simulink model "ashepwm_N3"  (R2017b)
settings: Solver=ode3  StartTime=0.0  StopTime=1  FixedStep=5e-6  MaxStep=1e-4  RelTol=1e-3
libraries: powerlib x12, simulink x1
settings Model: Creator=zsrx  LastModifiedBy=zsrx

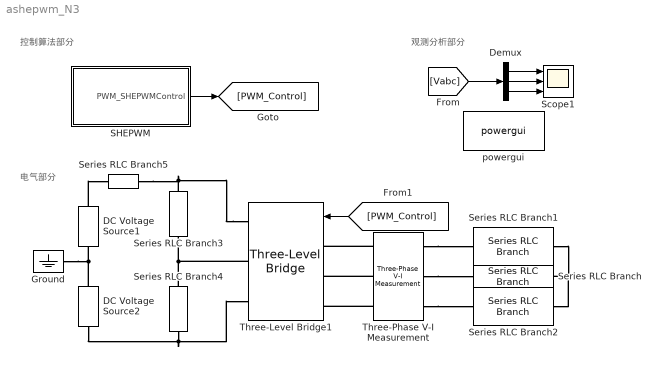
== system ashepwm_N3 ==
  note: 观测分析部分
  note: 控制算法部分
  note: 电气部分
  DC Voltage Source1 : powerlib/Electrical Sources/DC Voltage Source  Amplitude=345  Measurements=Voltage
  DC Voltage Source2 : powerlib/Electrical Sources/DC Voltage Source  Amplitude=345  Measurements=Voltage
  Demux : Demux  Outputs=3
  Ground : powerlib/Elements/Ground  LConnTagsString=a
  SHEPWM : Subsystem
  Scope1 : Scope  NumInputPorts=3
  Series RLC Branch : powerlib/Elements/Series RLC Branch  LConnTagsString=__new0  RConnTagsString=__new0  BranchType=R  Resistance=20  Inductance=1e-3  SetiL0=off  InitialCurrent=0  Capacitance=1e-6  Setx0=off  InitialVoltage=0  Measurements=None
  Series RLC Branch1 : powerlib/Elements/Series RLC Branch  LConnTagsString=__new0  RConnTagsString=__new0  BranchType=R  Resistance=20  Inductance=1e-3  SetiL0=off  InitialCurrent=0  Capacitance=1e-6  Setx0=off  InitialVoltage=0  Measurements=None
  Series RLC Branch2 : powerlib/Elements/Series RLC Branch  LConnTagsString=__new0  RConnTagsString=__new0  BranchType=R  Resistance=20  Inductance=1e-3  SetiL0=off  InitialCurrent=0  Capacitance=1e-6  Setx0=off  InitialVoltage=0  Measurements=None
  Series RLC Branch3 : powerlib/Elements/Series RLC Branch  LConnTagsString=__new0  RConnTagsString=__new0  BranchType=C  Resistance=20  Inductance=1e-3  SetiL0=off  InitialCurrent=0  Capacitance=9000e-6  Setx0=off  InitialVoltage=0  Measurements=None
  Series RLC Branch4 : powerlib/Elements/Series RLC Branch  LConnTagsString=__new0  RConnTagsString=__new0  BranchType=C  Resistance=20  Inductance=1e-3  SetiL0=off  InitialCurrent=0  Capacitance=9000e-6  Setx0=off  InitialVoltage=0  Measurements=None
  Series RLC Branch5 : powerlib/Elements/Series RLC Branch  LConnTagsString=__new0  RConnTagsString=__new0  BranchType=R  Resistance=0.001  Inductance=1e-3  SetiL0=off  InitialCurrent=0  Capacitance=1e-6  Setx0=off  InitialVoltage=0  Measurements=None
  Three-Level Bridge1 : powerlib/Power Electronics/Three-Level Bridge  Arms=3  SnubberResistance=1e5  SbubberCapacitance=inf  Device=GTO / Diodes  Ron=1e-3  ForwardVoltages="[  0  0  ]"  Measurements=None
      settings: SourceProductName=Simscape Power Systems  SourceProductBaseCode=PS
  Three-Phase V-I Measurement : powerlib/Measurements/Three-Phase V-I Measurement  VoltageMeasurement=phase-to-ground  SetLabelV=on  LabelV=Vabc  Vpu=off  VpuLL=off  CurrentMeasurement=yes  SetLabelI=on  LabelI=Iabc  Ipu=off  Pbase=100e6  Vbase=500e3  OutputType=Complex  PhasorSimulation=off  PSBequivalent=0
  powergui : powerlib/powergui  Priority=1  SimulationMode=Discrete  SampleTime=5e-6  frequency=60  Iterations=50  frequencyindice=0  Pbase=100e6  ErrMax=1e-4  UnitsV=kV  UnitsW=MW  buscounter=0  FunctionMessages=off  echomessages=off  EnableUseOfTLC=off  CurrentSourceSwitches=off  DisableSnubberDevices=off  DisableRonSwitches=off  DisableVfSwitches=off  DisplayEquations=off  SolverType=Tustin/Backward Euler (TBE)  Interpol=off  ExternalGateDelay=off  methode=off  Ts=100  x0status=blocks  SPID=off  SwTol=0  HookPort=off  RestoreLinks=warning  ResistiveCurrentMeasurement=off  Frange=[0:2:500]  Ylog=off  Xlog=on  ShowGrid=off  save=off  variable=ZData  structure=ScopeData1  ZoomFFT=off  StartTime=0.5  cycles=1  DisplayStyle=2  fundamental=50  FreqAxis=off  MaxFrequency=1000  frequencyindicesteady=1  RmsSteady=1  display=off
  wires:
  SHEPWM/1(PWM_SHEPWMControl) -> [PWM_Control]
  [PWM_Control] -> Three-Level Bridge1/1
  Demux/1 -> Scope1/1
  [Vabc] -> Demux/1
  Demux/2 -> Scope1/2
  Demux/3 -> Scope1/3
  connections:
  DC Voltage Source2/RConn1 -- Ground/LConn1 -- DC Voltage Source1/LConn1
  Three-Level Bridge1/RConn1 -- Series RLC Branch5/LConn1 -- Series RLC Branch3/LConn1
  DC Voltage Source2/LConn1 -- Series RLC Branch4/RConn1 -- Three-Level Bridge1/RConn3
  Series RLC Branch1/RConn1 -- Series RLC Branch2/RConn1 -- Series RLC Branch/RConn1
  Series RLC Branch4/LConn1 -- Three-Level Bridge1/RConn2 -- Series RLC Branch3/RConn1
  DC Voltage Source1/RConn1 -- Series RLC Branch5/RConn1
  Three-Phase V-I Measurement/LConn1 -- Three-Level Bridge1/LConn1
  Three-Phase V-I Measurement/LConn2 -- Three-Level Bridge1/LConn2
  Three-Phase V-I Measurement/LConn3 -- Three-Level Bridge1/LConn3
  Three-Phase V-I Measurement/RConn3 -- Series RLC Branch2/LConn1
  Three-Phase V-I Measurement/RConn2 -- Series RLC Branch/LConn1
  Three-Phase V-I Measurement/RConn1 -- Series RLC Branch1/LConn1

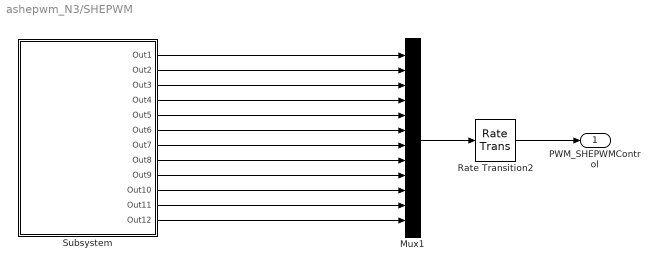
== system ashepwm_N3/SHEPWM ==
  Mux1 : Mux  Inputs=12
  Rate Transition2 : RateTransition  OutPortSampleTime=5e-6
  Subsystem : Subsystem
  PWM_SHEPWMControl : Outport
  wires:
  Subsystem/1(Out1) -> Mux1/1
  Subsystem/9(Out9) -> Mux1/9
  Subsystem/10(Out10) -> Mux1/10
  Subsystem/11(Out11) -> Mux1/11
  Subsystem/12(Out12) -> Mux1/12
  Mux1/1 -> Rate Transition2/1
  Subsystem/3(Out3) -> Mux1/3
  Subsystem/4(Out4) -> Mux1/4
  Subsystem/2(Out2) -> Mux1/2
  Subsystem/5(Out5) -> Mux1/5
  Subsystem/6(Out6) -> Mux1/6
  Subsystem/7(Out7) -> Mux1/7
  Subsystem/8(Out8) -> Mux1/8
  Rate Transition2/1 -> PWM_SHEPWMControl/1

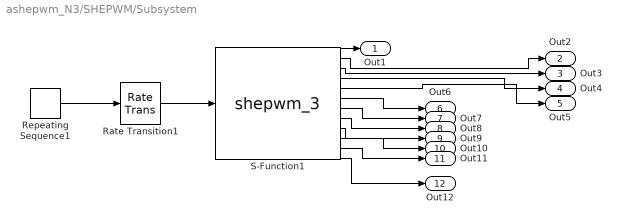
== system ashepwm_N3/SHEPWM/Subsystem ==
  Rate Transition1 : RateTransition  OutPortSampleTime=5e-5
  Repeating Sequence1 : simulink/Sources/Repeating Sequence  rep_seq_t=[0 0.02]  rep_seq_y=[0 6.2831852]
  S-Function1 : S-Function  FunctionName=shepwm_3  SFunctionDeploymentMode=off  EnableBusSupport=off
  Out1 : Outport
  Out2 : Outport  Port=2
  Out3 : Outport  Port=3
  Out4 : Outport  Port=4
  Out5 : Outport  Port=5
  Out6 : Outport  Port=6
  Out7 : Outport  Port=7
  Out8 : Outport  Port=8
  Out9 : Outport  Port=9
  Out10 : Outport  Port=10
  Out11 : Outport  Port=11
  Out12 : Outport  Port=12
  wires:
  S-Function1/1 -> Out1/1
  Repeating Sequence1/1 -> Rate Transition1/1
  Rate Transition1/1 -> S-Function1/1
  S-Function1/2 -> Out2/1
  S-Function1/4 -> Out4/1
  S-Function1/5 -> Out5/1
  S-Function1/3 -> Out3/1
  S-Function1/6 -> Out6/1
  S-Function1/7 -> Out7/1
  S-Function1/8 -> Out8/1
  S-Function1/9 -> Out9/1
  S-Function1/10 -> Out10/1
  S-Function1/11 -> Out11/1
  S-Function1/12 -> Out12/1
